simulink model "SimForcesGP2020a"  (R2020a)
settings: Solver=ode4  StartTime=0.0  StopTime=10  FixedStep=0.001  MaxStep=0.001  RelTol=1e-7
values from neighbouring files (symbols this model uses):
  B11_r_B11C = [0.23805608; 0.13201777; 0]    [InitializeSimulationGP.m]
  B11_r_B11Tc1 = [L11; 0; 0]    [InitializeSimulationGP.m]
  B11_Rot_Tc1 = eye(3)    [InitializeSimulationGP.m]
  B11cI = [0.28426000 -0.06487287 0;         -0.06487287  0.54237481 0;                   0  0          0.67891020]    [InitializeSimulationGP.m]
  B12_r_B12C = [0.60504569; 0.27199376; 0.00002484]    [InitializeSimulationGP.m]
  B12_r_B12Tc2 = [L12;0;0]    [InitializeSimulationGP.m]
  B12_Rot_Tc2 = eye(3)    [InitializeSimulationGP.m]
  B12cI = [1.18803886 -2.36786418 0.00280315;          -2.36786418 6.31493281 0.00022322;           0.00280315 0.00022322 7.40915161]    [InitializeSimulationGP.m]
  B31_r_B31C = [0.35781210 0 0]    [InitializeSimulationGP.m]
  B31_Rot_B41 = eye(3)    [InitializeSimulationGP.m]
  B31cI = diag([0.03150902 0.90735702 0.90763033])    [InitializeSimulationGP.m]
  B32_r_B32C = [0.35781210 0 0]    [InitializeSimulationGP.m]
  B32_Rot_B42 = eye(3)    [InitializeSimulationGP.m]
  B32cI = diag([0.03150902 0.90735702 0.90763033])    [InitializeSimulationGP.m]
  B41_r_B41C = [0.55785997 0 0]    [InitializeSimulationGP.m]
  B41_r_B41Tc1 = [lc1;0;0]    [InitializeSimulationGP.m]
  B41cI = diag([0.00370720 0.55759812 0.55785997])    [InitializeSimulationGP.m]
  B42_r_B42C = [0.55785997 0 0]    [InitializeSimulationGP.m]
  B42_r_B42Tc2 = [lc2; 0; 0]    [InitializeSimulationGP.m]
  B42cI = diag([0.00370720 0.55759812 0.55785997])    [InitializeSimulationGP.m]
  B52_r_B52C = [0 0 0.56802906]    [InitializeSimulationGP.m]
  B52_r_B52P32 = [lc3; 0; 0]    [InitializeSimulationGP.m]
  B52_Rot_P32 = eye(3)    [InitializeSimulationGP.m]
  B52cI = diag([0.91789884, 0.91790043, 0.00091463])    [InitializeSimulationGP.m]
  Bc1_r_Bc1B11 = [L1; 0; 0]    [InitializeSimulationGP.m]
  Bc1_r_Bc1B31 = [0;0;0]    [InitializeSimulationGP.m]
  Bc1_r_Bc1C = [0.14178771; 0.16555780; 0]    [InitializeSimulationGP.m]
  Bc1_V = [0;0;0;0;0;0]    [InitializeSimulationGP.m]
  Bc1cI = [+5.892211080 +5.476111360 -0.000019630;          +5.476111360 +28.66965601 -0.000024550;          -0.000019630 -0.000024550 +29.78955950]    [InitializeSimulationGP.m]
  Bc2_r_Bc2B12 = [L2;0;0]    [InitializeSimulationGP.m]
  Bc2_r_Bc2B32 = [0;0;0]    [InitializeSimulationGP.m]
  Bc2_r_Bc2C = [0.54319901; 0.10543875; 0]    [InitializeSimulationGP.m]
  Bc2cI = [0.48071390 0.52924041 0;          0.52924041 5.80912352 0;              0      0          5.97255351]    [InitializeSimulationGP.m]
  beta1 = atan2d(374.261,935)*pi/180    [InitializeSimulationGP.m]
  beta2 = atan2d(45.757,373.313)*pi/180    [InitializeSimulationGP.m]
  beta3 = atan2d(139.50,1132.19)*pi/180    [InitializeSimulationGP.m]
  beta4 = atan2d(88.061,296.198)*pi/180    [InitializeSimulationGP.m]
  D22F = [0;0;0;0;0;0]    [InitializeSimulationGP.m]
  L1 = 1.0071227324212    (= 1.00712273242)    [InitializeSimulationGP.m]
  L11 = 0.37610632101293    (= 0.376106321013)    [InitializeSimulationGP.m]
  L12 = 0.30901132665325    (= 0.309011326653)    [InitializeSimulationGP.m]
  L2 = 1.132185817991    (= 1.13218581799)    [InitializeSimulationGP.m]
  lc1 = 0.745    [InitializeSimulationGP.m]
  lc2 = 0.745    [InitializeSimulationGP.m]
  mB11 = 25.52660174    [InitializeSimulationGP.m]
  mB12 = 33.92850233    [InitializeSimulationGP.m]
  mB31 = 17.36281648    [InitializeSimulationGP.m]
  mB32 = 17.36281648    [InitializeSimulationGP.m]
  mB41 = 10.34519231    [InitializeSimulationGP.m]
  mB42 = 10.34519231    [InitializeSimulationGP.m]
  mB52 = 6.73059863    [InitializeSimulationGP.m]
  mBc1 = 307.29601379    [InitializeSimulationGP.m]
  mBc2 = 54.58702836    [InitializeSimulationGP.m]
  mP22 = 9.26136143    [InitializeSimulationGP.m]
  mP32 = 570.18877059    [InitializeSimulationGP.m]
  P22_r_P22C = [0.62192523 0 0]    [InitializeSimulationGP.m]
  P22_Rot_B52 = eye(3)    [InitializeSimulationGP.m]
  P22cI = diag([0.00662754, 1.48387017, 1.48398069])    [InitializeSimulationGP.m]
  P32_r_P32C = [0.25466704; -0.13034397; -0.01302248]    [InitializeSimulationGP.m]
  P32_r_P32D22 = [0.40499744871392; -0.13130517281345; -0.013385243295654]    [InitializeSimulationGP.m]
  P32_Rot_D22 = [1 0 0;              0 0.9707729441837 0.23999977258512;              0 -0.23999977258512 0.9707729441837]    [InitializeSimulationGP.m]
  P32cI = [46.81220713 0.38607676 -0.00453819;          0.38607676 71.92201786 -1.14320993;          -0.00453819 -1.14320993 67.38128576]    [InitializeSimulationGP.m]
  Tc1_r_Tc1Bc2 = [0.098495302558553; 0.01838181329939; 0]    [InitializeSimulationGP.m]
  Tc1_Rot_Bc2 = [cos(alpha2) -sin(alpha2) 0;                sin(alpha2)  cos(alpha2) 0;                0            0           1]    [InitializeSimulationGP.m]
  Tc2_r_Tc2P22 = [-0.048858374920227;0.36587359346146;0.035276938723102]    [InitializeSimulationGP.m]
  Tc2_Rot_P22 = [0.95853460763586 -0.27664713597974  0.0683942111482;                0.28497614981675  0.93051946315663 -0.23004808784757;                0                 0.23999977258511  0.9707729441837]    [InitializeSimulationGP.m]
  Th1A = 5*pi/180    (= 0.0872664625997)    [InitializeSimulationGP.m]
  Th1B = 20*pi/180    (= 0.349065850399)    [InitializeSimulationGP.m]
  Th1f = 1    [InitializeSimulationGP.m]
  Th2A = 15*pi/180    (= 0.261799387799)    [InitializeSimulationGP.m]
  Th2B = -50*pi/180    (= -0.872664625997)    [InitializeSimulationGP.m]
  Th2f = 2    [InitializeSimulationGP.m]
  W_r_WBc1 = [0.185;-0.085;0]    [InitializeSimulationGP.m]
  W_Rot_Bc1 = [cos(alpha1) -sin(alpha1) 0;              sin(alpha1)  cos(alpha1) 0;              0            0           1]    [InitializeSimulationGP.m]
  Wg = [0; 9.8066; 0]    [InitializeSimulationGP.m]
  x10 = 0.83    [InitializeSimulationGP.m]
  x20 = 0.83    [InitializeSimulationGP.m]
  x3A = 0.1    [InitializeSimulationGP.m]
  x3B = 0.5    [InitializeSimulationGP.m]
  x3f = 1    [InitializeSimulationGP.m]
  xf = [1;0;0;0;0;0]    [InitializeSimulationGP.m]
  ztau = [0;0;0;0;0;1]    [InitializeSimulationGP.m]
undefined symbols (not defined in the file or in its folder): B11_V, B11_V_SS, B11Ftot, B12_U_Tc2, B12_V, B12_V_SS, B12Ftot, B31_r_B31B41, B31_V, B31_V_SS, B31FTot, B32_r_B32B42, B32_U_B42, B32_V, B32_V_SS, B32FTot, B41_V, B41_V_SS, B41FTot, B42_Rot_Tc2, B42_U_Tc2, B42_V, B42_V_SS, B42FTot, B52_U_P32, B52_V, B52_V_SS, B52Ftot, Bc1_V_SS, Bc1Tot, Bc2_Rot_B12, Bc2_Rot_B32, Bc2_U_B12, Bc2_U_B32, Bc2_V, Bc2_V_SS, Bc2Tot, D22_V, D22_V_SS, dq1, dq11, dq12, dq2, dq21, dq22, dx1, dx2, FTot_S1, FTot_S2P, FTot_S2R, P22_r_P22B52, P22_U_B52, P22_V, P22_V_SS, P22FTot, P32_U_D22, P32_V, P32_V_SS, P32FTot, q1 ... (+28)
libraries: nesl_utility x94, sm_lib x45
(part 4 of 6)

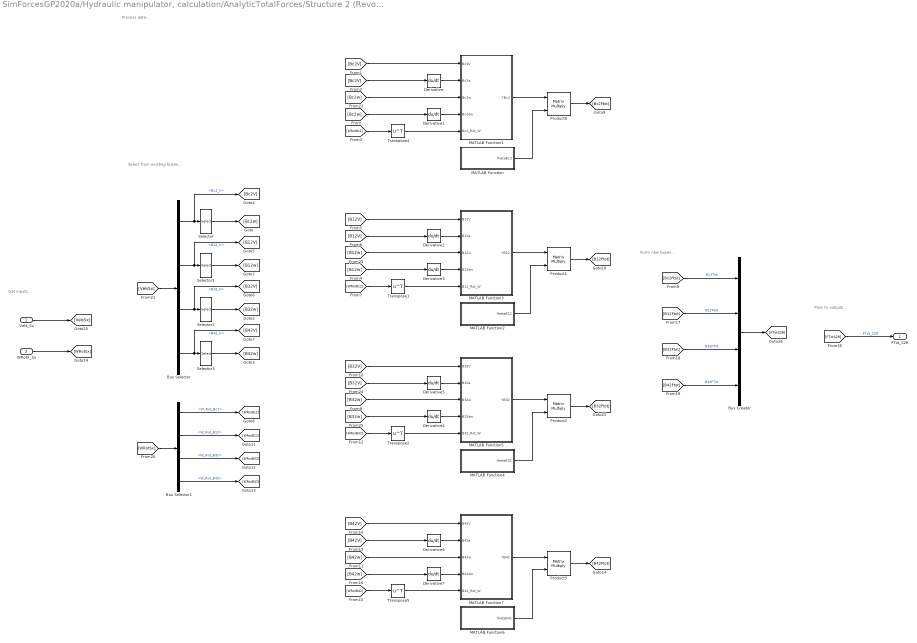
== system SimForcesGP2020a/Hydraulic manipulator, calculation/AnalyticTotalForces/Structure 2 (Revolute segment) ==
  note: Process data...
  note: Pass to outputs...
  note: Get inputs...
  note: Form new buses...
  note: Select from existing buses...
  Vels_Sx : Inport
  WRotX_Sx : Inport  Port=2
  Bus Creator : BusCreator  Inputs=Bc2Tot,B12Ftot,B32FTot,B42FTot
  Bus Selector : BusSelector  OutputSignals=Vels_S1.Bc2_V,Vels_S2R.B12_V,Vels_S2R.B32_V,Vels_S2R.B42_V
  Bus Selector1 : BusSelector  OutputSignals=WRotX_S1.W_Rot_Bc2,WRotX_S2R.W_Rot_B12,WRotX_S2R.W_Rot_B32,WRotX_S2R.W_Rot_B42
  Derivative{,1..7} (8 alike) : Derivative
  MATLAB Function : MATLAB Function  TreatAsAtomicUnit=on
  MATLAB Function1 : MATLAB Function  TreatAsAtomicUnit=on
  MATLAB Function2 : MATLAB Function  TreatAsAtomicUnit=on
  MATLAB Function3 : MATLAB Function  TreatAsAtomicUnit=on
  MATLAB Function4 : MATLAB Function  TreatAsAtomicUnit=on
  MATLAB Function5 : MATLAB Function  TreatAsAtomicUnit=on
  MATLAB Function6 : MATLAB Function  TreatAsAtomicUnit=on
  MATLAB Function7 : MATLAB Function  TreatAsAtomicUnit=on
  Product{1..3,8} (4 alike) : Product  Multiplication=Matrix(*)
  Selector{,1..3} (4 alike) : Selector  InputPortWidth=6  IndexOptions=Index vector (dialog)  Indices=[4 5 6]  OutputSizes=1
  Transpose{1..2,4..5} (4 alike) : Math  Operator=transpose  SaturateOnIntegerOverflow=on
  FTot_S2R : Outport
  wires:
  Bus Selector1/4 -> [WRotB42]  "<W_Rot_B42>"
  [WRotB12] -> Transpose1/1
  Bus Selector1/2 -> [WRotB12]  "<W_Rot_B12>"
  [WRotB42] -> Transpose5/1
  [Bc2Ftot] -> Bus Creator/1  "Bc2Tot"
  Selector2/1 -> [B32w]
  [B42Ftot] -> Bus Creator/4  "B42FTot"
  Bus Selector/2 -> Selector1/1, [B12V]  "<B12_V>"
  Bus Selector/1 -> Selector/1, [Bc2V]  "<Bc2_V>"
  [B32Ftot] -> Bus Creator/3  "B32FTot"
  Bus Selector/3 -> Selector2/1, [B32V]  "<B32_V>"
  Selector1/1 -> [B12w]
  [WRotSx] -> Bus Selector1/1
  Selector3/1 -> [B42w]
  Bus Creator/1 -> [FTotS2R]
  Selector/1 -> [Bc2w]
  [WRotB32] -> Transpose2/1
  Product3/1 -> [B42Ftot]
  Product8/1 -> [Bc2Ftot]
  [B12Ftot] -> Bus Creator/2  "B12Ftot"
  Bus Selector1/1 -> [WRotBc2]  "<W_Rot_Bc2>"
  [VelsSx] -> Bus Selector/1
  Bus Selector1/3 -> [WRotB32]  "<W_Rot_B32>"
  Bus Selector/4 -> Selector3/1, [B42V]  "<B42_V>"
  Vels_Sx/1 -> [VelsSx]
  WRotX_Sx/1 -> [WRotSx]
  [FTotS2R] -> FTot_S2R/1  "FTot_S2R"
  [Bc2w] -> Derivative1/1
  [Bc2w] -> MATLAB Function1/3(Bc2w)
  [WRotBc2] -> Transpose4/1
  Transpose4/1 -> MATLAB Function1/5(Bc2_Rot_W)
  Derivative1/1 -> MATLAB Function1/4(Bc2dw)
  [Bc2V] -> MATLAB Function1/1(Bc2V)
  MATLAB Function/1(thetaBc2) -> Product8/2
  [Bc2V] -> Derivative/1
  MATLAB Function1/1(YBc2) -> Product8/1
  Derivative/1 -> MATLAB Function1/2(Bc2a)
  Derivative2/1 -> MATLAB Function3/2(B12a)
  MATLAB Function3/1(YB12) -> Product1/1
  [B12V] -> Derivative2/1
  MATLAB Function2/1(thetaB12) -> Product1/2
  [B12V] -> MATLAB Function3/1(B12V)
  Derivative3/1 -> MATLAB Function3/4(B12dw)
  Transpose1/1 -> MATLAB Function3/5(B12_Rot_W)
  [B12w] -> MATLAB Function3/3(B12w)
  [B12w] -> Derivative3/1
  Product1/1 -> [B12Ftot]
  [B32w] -> Derivative4/1
  [B32w] -> MATLAB Function5/3(B32w)
  Derivative4/1 -> MATLAB Function5/4(B32dw)
  [B32V] -> MATLAB Function5/1(B32V)
  MATLAB Function4/1(thetaB32) -> Product2/2
  [B32V] -> Derivative5/1
  MATLAB Function5/1(YB32) -> Product2/1
  Derivative5/1 -> MATLAB Function5/2(B32a)
  Transpose2/1 -> MATLAB Function5/5(B32_Rot_W)
  Product2/1 -> [B32Ftot]
  Transpose5/1 -> MATLAB Function7/5(B42_Rot_W)
  Derivative6/1 -> MATLAB Function7/2(B42a)
  MATLAB Function7/1(YB42) -> Product3/1
  [B42V] -> Derivative6/1
  MATLAB Function6/1(thetaB42) -> Product3/2
  [B42V] -> MATLAB Function7/1(B42V)
  Derivative7/1 -> MATLAB Function7/4(B42dw)
  [B42w] -> MATLAB Function7/3(B42w)
  [B42w] -> Derivative7/1

== system SimForcesGP2020a/Hydraulic manipulator, calculation/AnalyticVelocities/Structure 1 ==
  note: Pass to outputs...
  note: Process data...
  note: Calculate geometric properties of the closed kinematic chain 1...
  note: Get inputs...
  note: Form relevant position vectors...
  note: Form relevant rotation matrices...
  note: Form relevant velocity/force transformation matrices...
  note: Form relevant linear/angular velocities...
  q1[rad] : Inport  Unit=rad
  W_Rot_Bc1 : Inport  Port=2
  Bc1_V : Inport  Port=3  PortDimensions=[6 1]
  GeomPropS1 : Subsystem
  PosVecsS1 : Subsystem
  RotMatsS1 : Subsystem
  UMatsS1 : Subsystem
  VelsS1 : Subsystem
  Geom_S1 : Outport
  PosVecs_S1 : Outport  Port=2
  WRotX_S1 : Outport  Port=3
  Vels_S1 : Outport  Port=4
  UMat_S1 : Outport  Port=5
  wires:
  GeomPropS1/1(GeomProp_S1) -> [GeomS1]
  [GeomS1] -> PosVecsS1/1(GeomProp_CC1)
  [GeomS1] -> RotMatsS1/1(GeomProp_S1)
  [GeomS1] -> VelsS1/1(GeomProp_S1)
  RotMatsS1/1(RotMats_S1) -> [RotMatsS1]
  [RotMatsS1] -> UMatsS1/2(RotMats_S1)
  PosVecsS1/1(PosVecs_S1) -> [PosVecsS1]
  [PosVecsS1] -> UMatsS1/1(PosVecs_S1)
  [GeomS1] -> Geom_S1/1
  VelsS1/1(Vels_S1) -> [VelsS1]
  [VelsS1] -> Vels_S1/1
  UMatsS1/1(UMat_S1) -> [UMatsS1]
  [UMatsS1] -> VelsS1/2(UMats_S1)
  Bc1_V/1 -> [Bc1V]  "Bc1V"
  [Bc1V] -> VelsS1/3(Bc1_V)
  W_Rot_Bc1/1 -> [WRotBc1]  "WRotBc1"
  [WRotBc1] -> RotMatsS1/2(WRotBc1)
  [UMatsS1] -> UMat_S1/1
  RotMatsS1/2(WRotX_S1) -> [WRotXS1]
  [WRotXS1] -> WRotX_S1/1
  q1[rad]/1 -> [q1]  "q1"
  [q1] -> GeomPropS1/1(q1)
  [PosVecsS1] -> PosVecs_S1/1

== system SimForcesGP2020a/Hydraulic manipulator, calculation/AnalyticVelocities/Structure 2 (Prismatic segment) ==
  note: Pass to outputs...
  note: Get inputs...
  note: Process data...
  x3 : Inport
  WRotX_S2R : Inport  Port=2
  Vels_S2R : Inport  Port=3
  GeomPropS2P : Subsystem
  PosVecsS2P : Subsystem
  RotMatsS2P : Subsystem
  UMatsS2P : Subsystem
  VelsS2P : Subsystem
  GeomProp_S2P : Outport
  PosVecs_S2P : Outport  Port=2
  WRotX_S2P : Outport  Port=3
  Vels_S2P : Outport  Port=4
  UMats_S2P : Outport  Port=5
  wires:
  x3/1 -> [x3]
  Vels_S2R/1 -> [VelsS2R]
  WRotX_S2R/1 -> [WRotXS2R]
  GeomPropS2P/1(GeomProp_S2P) -> [GeomS2P]
  [GeomS2P] -> GeomProp_S2P/1
  [x3] -> GeomPropS2P/1(x3)
  PosVecsS2P/1(PosVecsS2P) -> [PosVecsS2P]
  [x3] -> PosVecsS2P/1(x3)
  [PosVecsS2P] -> PosVecs_S2P/1
  RotMatsS2P/2(WRotX_S2P) -> [WRotXS2P]
  [WRotXS2R] -> RotMatsS2P/1(WRotX_S2R)
  [WRotXS2P] -> WRotX_S2P/1
  RotMatsS2P/1(RotMats_S2P) -> [RotMatsS2P]
  [PosVecsS2P] -> UMatsS2P/1(PosVecs_S2P)
  [RotMatsS2P] -> UMatsS2P/2(RotMats_S2P)
  UMatsS2P/1(UMats_S2P) -> [UMatsS2P]
  [UMatsS2P] -> UMats_S2P/1
  [VelsS2R] -> VelsS2P/3(Vels_S2R)
  [GeomS2P] -> VelsS2P/1(GeomProp_S2P)
  [UMatsS2P] -> VelsS2P/2(UMats_S2P)
  VelsS2P/1(Vels_S2P) -> [VelsS2P]
  [VelsS2P] -> Vels_S2P/1

== system SimForcesGP2020a/Hydraulic manipulator, calculation/AnalyticVelocities/Structure 2 (Revolute segment) ==
  note: Pass to outputs...
  note: Process data...
  note: Get inputs...
  q2[rad] : Inport
  WRotX_S1 : Inport  Port=2
  Vels_S1 : Inport  Port=3
  GeomPropS2R : Subsystem
  PosVecsS2R : Subsystem
  RotMatsS2R : Subsystem
  UMatS2R : Subsystem
  VelsS2R : Subsystem
  GeomProp_S2R : Outport
  PosVecs_S2R : Outport  Port=2
  WRotX_S2R : Outport  Port=3
  Vels_S2R : Outport  Port=4
  UMats_S2R : Outport  Port=5
  wires:
  [GeomS2R] -> VelsS2R/1(GeomProp_CC2)
  [GeomS2R] -> RotMatsS2R/1(GeomProp_CC2)
  [GeomS2R] -> PosVecsS2R/1(GeomProp_S2R)
  GeomPropS2R/1(GeomProp_S2R) -> [GeomS2R]
  [q2] -> GeomPropS2R/1(q2)
  [GeomS2R] -> GeomProp_S2R/1  "GeomS2R"
  RotMatsS2R/1(RotMats_S2) -> [RotMatsS2R]
  q2[rad]/1 -> [q2]  "q2"
  PosVecsS2R/1(PosVecs_S2) -> [PosVecsS2R]
  [PosVecsS2R] -> UMatS2R/1(PosVecs_S2)
  [PosVecsS2R] -> PosVecs_S2R/1  "PosVecsS2R"
  [RotMatsS2R] -> UMatS2R/2(RotMats_S2)
  UMatS2R/1(UMatS2) -> [UMatsS2R]
  [UMatsS2R] -> VelsS2R/2(UMats_S2)
  [UMatsS2R] -> UMats_S2R/1  "UMatsS2R"
  RotMatsS2R/2(WRotX_S2) -> [WRotXS2R]
  [WRotXS2R] -> WRotX_S2R/1  "WRotXS2R"
  Vels_S1/1 -> [VelsS1]  "Vels_S1"
  [VelsS1] -> VelsS2R/3(Vels_S1)
  WRotX_S1/1 -> [WRotXS1]  "WRotX_S1"
  [WRotXS1] -> RotMatsS2R/2(WRotX_S1)
  VelsS2R/1(Vels_S2) -> [VelsS2R]
  [VelsS2R] -> Vels_S2R/1  "VelsS2R"

== system SimForcesGP2020a/Hydraulic manipulator, calculation/AnalyticVelocities/Structure 1/GeomPropS1 ==
  note: Get inputs...
  note: Pass to outputs...
  note: Process data...
  note: Create new buses...
  q1 : Inport
  Bus Creator : BusCreator  Inputs=q1,x1,q11,q12,dq1,dx1,dq11,dq12
  LiftPistonStroke : Subsystem
  Subsystem : Subsystem
  Subsystem1 : Subsystem
  Subsystem2 : Subsystem
  q11-angle : Subsystem
  q12-angle : Subsystem
  q1Derivative : Subsystem
  GeomProp_S1 : Outport
  wires:
  q1/1 -> [q1]  "q1"
  [q1] -> LiftPistonStroke/1(q1[rad])  "q1"
  LiftPistonStroke/1(x1[m]) -> [x1]  "x1"
  [x1] -> q11-angle/1(x1)  "x1"
  [x1] -> q12-angle/1(x1)  "x1"
  [dq1] -> Bus Creator/5  "dq1"
  q12-angle/1(q12) -> [q12]  "q12"
  [q12] -> Bus Creator/4  "q12"
  [q1] -> Bus Creator/1  "q1"
  [x1] -> Bus Creator/2  "x1"
  q11-angle/1(q11) -> [q11]  "q11"
  [q11] -> Bus Creator/3  "q11"
  [dx1] -> Bus Creator/6  "dx1"
  [dq12] -> Bus Creator/8  "dq12"
  [dq11] -> Bus Creator/7  "dq11"
  Bus Creator/1 -> [GeomPropS1]
  [GeomPropS1] -> GeomProp_S1/1
  [q1] -> q1Derivative/1(q1)  "q1"
  q1Derivative/1(dq1) -> [dq1]  "dq1"
  [dq1] -> Subsystem/1(dq1)  "dq1"
  [x1] -> Subsystem/2(x1)  "x1"
  [q1] -> Subsystem/3(q1)  "q1"
  Subsystem/1(dx1) -> [dx1]  "dx1"
  [dx1] -> Subsystem1/3(dx1)  "dx1"
  [x1] -> Subsystem1/1(x1)  "x1"
  [q11] -> Subsystem1/2(q11)  "q11"
  Subsystem1/1(dq11) -> [dq11]  "dq11"
  Subsystem2/1(dq12) -> [dq12]  "dq12"
  [dx1] -> Subsystem2/3(dx1)  "dx1"
  [x1] -> Subsystem2/1(x1)  "x1"
  [q12] -> Subsystem2/2(q12)  "q12"

== system SimForcesGP2020a/Hydraulic manipulator, calculation/AnalyticVelocities/Structure 1/PosVecsS1 ==
  note: Select from existing buses...
  note: Pass to outputs...
  note: Create new buses...
  note: Process data...
  note: Form time-varying position vectors...
  note: Get inputs...
  GeomProp_CC1 : Inport
  B11_r_B11Tc1 : Constant  Value=B11_r_B11Tc1
  B31_r_B31B41 : MATLAB Function  TreatAsAtomicUnit=on
  B41_r_B41Tc1 : Constant  Value=B41_r_B41Tc1
  Bc1_r_Bc1B1 : Constant  Value=W_r_WBc1
  Bc1_r_Bc1B11 : Constant  Value=Bc1_r_Bc1B11
  Bc1_r_Bc1B31 : Constant  Value=Bc1_r_Bc1B31
  Bus Creator : BusCreator  Inputs=Tc1_r_Tc1Bc2,B41_r_B41Tc1,B31_r_B31B41,Bc1_r_Bc1B31,B11_r_B11Tc1,Bc1_r_Bc1B11,W_r_WBc1
  Bus Selector : BusSelector  OutputSignals=x1
  Tc1_r_Tc1Bc2 : Constant  Value=Tc1_r_Tc1Bc2
  PosVecs_S1 : Outport
  wires:
  Bus Creator/1 -> [PosVecsS1]
  GeomProp_CC1/1 -> [GeomPropCC1]  "GeomProp_CC1"
  [GeomPropCC1] -> Bus Selector/1
  Tc1_r_Tc1Bc2/1 -> [rTc1Bc2]  "Tc1_r_Tc1Bc2"
  [rTc1Bc2] -> Bus Creator/1  "Tc1_r_Tc1Bc2"
  B41_r_B41Tc1/1 -> [rB41Tc1]  "B41_r_B41Tc1"
  [rB41Tc1] -> Bus Creator/2  "B41_r_B41Tc1"
  B31_r_B31B41/1(B31_r_B31B41) -> [rB31B41]  "B31_r_B31B41"
  [rB31B41] -> Bus Creator/3  "B31_r_B31B41"
  Bc1_r_Bc1B31/1 -> [rBc1B31]  "Bc1_r_Bc1B31"
  B11_r_B11Tc1/1 -> [rB11Tc1]  "B11_r_B11Tc1"
  Bc1_r_Bc1B11/1 -> [rBc1B11]  "Bc1_r_Bc1B11"
  [rBc1B31] -> Bus Creator/4  "Bc1_r_Bc1B31"
  [rB11Tc1] -> Bus Creator/5  "B11_r_B11Tc1"
  [rBc1B11] -> Bus Creator/6  "Bc1_r_Bc1B11"
  Bus Selector/1 -> [x1]  "<x1>"
  [x1] -> B31_r_B31B41/1(x1)
  [PosVecsS1] -> PosVecs_S1/1  "PosVecs_S1"
  [rWBc1] -> Bus Creator/7  "W_r_WBc1"
  Bc1_r_Bc1B1/1 -> [rWBc1]  "W_r_WBc1"

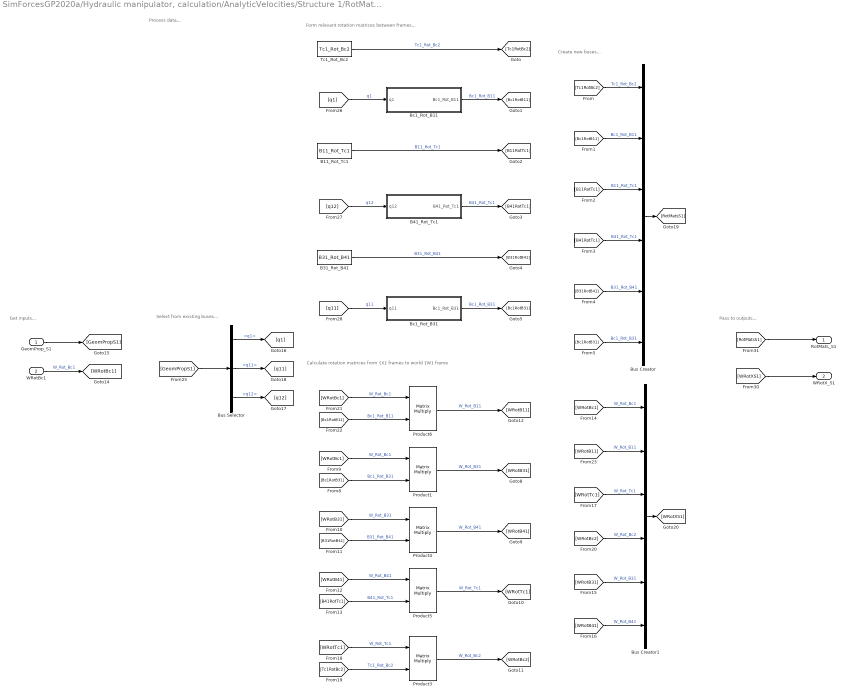
== system SimForcesGP2020a/Hydraulic manipulator, calculation/AnalyticVelocities/Structure 1/RotMatsS1 ==
  note: Create new buses...
  note: Pass to outputs...
  note: Get inputs...
  note: Process data...
  note: Select from existing buses...
  note: Form relevant rotation matrices between frames...
  note: Calculate rotation matrices from {X} frames to world {W} frame
  GeomProp_S1 : Inport
  WRotBc1 : Inport  Port=2
  B11_Rot_Tc1 : Constant  Value=B11_Rot_Tc1
  B31_Rot_B41 : Constant  Value=B31_Rot_B41
  B41_Rot_Tc1 : MATLAB Function  TreatAsAtomicUnit=on
  Bc1_Rot_B11 : MATLAB Function  TreatAsAtomicUnit=on
  Bc1_Rot_B31 : MATLAB Function  TreatAsAtomicUnit=on
  Bus Creator : BusCreator  Inputs=6
  Bus Creator1 : BusCreator  Inputs=W_Rot_Bc1,W_Rot_B11,W_Rot_Tc1,W_Rot_Bc2,W_Rot_B31,W_Rot_B41
  Bus Selector : BusSelector  OutputSignals=q1,q11,q12
  Product{1,3..6} (5 alike) : Product  Multiplication=Matrix(*)
  Tc1_Rot_Bc2 : Constant  Value=Tc1_Rot_Bc2
  RotMats_S1 : Outport
  WRotX_S1 : Outport  Port=2
  wires:
  [Tc1RotBc2] -> Bus Creator/1  "Tc1_Rot_Bc2"
  Tc1_Rot_Bc2/1 -> [Tc1RotBc2]  "Tc1_Rot_Bc2"
  [Bc1RotB11] -> Bus Creator/2  "Bc1_Rot_B11"
  Bc1_Rot_B11/1(Bc1_Rot_B11) -> [Bc1RotB11]  "Bc1_Rot_B11"
  [B11RotTc1] -> Bus Creator/3  "B11_Rot_Tc1"
  B11_Rot_Tc1/1 -> [B11RotTc1]  "B11_Rot_Tc1"
  B41_Rot_Tc1/1(B41_Rot_Tc1) -> [B41RotTc1]  "B41_Rot_Tc1"
  [B41RotTc1] -> Bus Creator/4  "B41_Rot_Tc1"
  B31_Rot_B41/1 -> [B31RotB41]  "B31_Rot_B41"
  [B31RotB41] -> Bus Creator/5  "B31_Rot_B41"
  Bc1_Rot_B31/1(Bc1_Rot_B31) -> [Bc1RotB31]  "Bc1_Rot_B31"
  [Bc1RotB31] -> Bus Creator/6  "Bc1_Rot_B31"
  [WRotBc1] -> Product1/1  "W_Rot_Bc1"
  [Bc1RotB31] -> Product1/2  "Bc1_Rot_B31"
  Product1/1 -> [WRotB31]  "W_Rot_B31"
  [WRotB31] -> Product4/1  "W_Rot_B31"
  [B31RotB41] -> Product4/2  "B31_Rot_B41"
  Product4/1 -> [WRotB41]  "W_Rot_B41"
  Product5/1 -> [WRotTc1]  "W_Rot_Tc1"
  [B41RotTc1] -> Product5/2  "B41_Rot_Tc1"
  [WRotB41] -> Product5/1  "W_Rot_B41"
  [WRotTc1] -> Product3/1  "W_Rot_Tc1"
  [Tc1RotBc2] -> Product3/2  "Tc1_Rot_Bc2"
  Product3/1 -> [WRotBc2]  "W_Rot_Bc2"
  [WRotBc1] -> Product6/1  "W_Rot_Bc1"
  [Bc1RotB11] -> Product6/2  "Bc1_Rot_B11"
  Product6/1 -> [WRotB11]  "W_Rot_B11"
  [WRotB11] -> Bus Creator1/2  "W_Rot_B11"
  [WRotBc1] -> Bus Creator1/1  "W_Rot_Bc1"
  [WRotB41] -> Bus Creator1/6  "W_Rot_B41"
  [WRotB31] -> Bus Creator1/5  "W_Rot_B31"
  [WRotBc2] -> Bus Creator1/4  "W_Rot_Bc2"
  [WRotTc1] -> Bus Creator1/3  "W_Rot_Tc1"
  WRotBc1/1 -> [WRotBc1]  "W_Rot_Bc1"
  GeomProp_S1/1 -> [GeomPropS1]
  [GeomPropS1] -> Bus Selector/1
  Bus Selector/1 -> [q1]  "<q1>"
  Bus Selector/3 -> [q12]  "<q12>"
  Bus Selector/2 -> [q11]  "<q11>"
  [q1] -> Bc1_Rot_B11/1(q1)  "q1"
  [q12] -> B41_Rot_Tc1/1(q12)  "q12"
  [q11] -> Bc1_Rot_B31/1(q11)  "q11"
  Bus Creator/1 -> [RotMatsS1]
  Bus Creator1/1 -> [WRotXS1]
  [WRotXS1] -> WRotX_S1/1
  [RotMatsS1] -> RotMats_S1/1

== system SimForcesGP2020a/Hydraulic manipulator, calculation/AnalyticVelocities/Structure 1/UMatsS1 ==
  note: Get inputs...
  note: Pass to outputs...
  note: Form new buses...
  note: Process data...
  note: Form relevant velocity/force transformation matrices...
  note: Select form existing buses...
  PosVecs_S1 : Inport
  RotMats_S1 : Inport  Port=2
  B11_U_Tc1 : MATLAB Function  TreatAsAtomicUnit=on
  B31_U_B41 : MATLAB Function  TreatAsAtomicUnit=on
  B41_U_Tc1 : MATLAB Function  TreatAsAtomicUnit=on
  Bc1_U_B11 : MATLAB Function  TreatAsAtomicUnit=on
  Bc1_U_B31 : MATLAB Function  TreatAsAtomicUnit=on
  Bus Creator : BusCreator  Inputs=6
  Bus Selector : BusSelector  OutputSignals=Tc1_r_Tc1Bc2,B41_r_B41Tc1,B31_r_B31B41,Bc1_r_Bc1B31,B11_r_B11Tc1,Bc1_r_Bc1B11
  Bus Selector1 : BusSelector  OutputSignals=Tc1_Rot_Bc2,B41_Rot_Tc1,B31_Rot_B41,Bc1_Rot_B31,B11_Rot_Tc1,Bc1_Rot_B11
  Tc1_U_Bc2 : MATLAB Function  TreatAsAtomicUnit=on
  UMat_S1 : Outport
  wires:
  Bus Selector/2 -> [rB41Tc1]  "<B41_r_B41Tc1>"
  [rB41Tc1] -> B41_U_Tc1/1(B41_r_B41Tc1)
  Bus Selector/3 -> [rB31B41]  "<B31_r_B31B41>"
  Bus Selector/5 -> [rB11Tc1]  "<B11_r_B11Tc1>"
  Bus Selector/4 -> [rBc1B31]  "<Bc1_r_Bc1B31>"
  Bus Selector/6 -> [rBc1B11]  "<Bc1_r_Bc1B11>"
  [rBc1B11] -> Bc1_U_B11/1(Bc1_r_Bc1B11)
  [rB11Tc1] -> B11_U_Tc1/1(B11_r_B11Tc1)
  [rBc1B31] -> Bc1_U_B31/1(Bc1_r_Bc1B31)
  [rB31B41] -> B31_U_B41/1(B31_r_B31B41)
  Bus Selector1/2 -> [B41RotTc1]  "<B41_Rot_Tc1>"
  Bus Selector1/3 -> [B31RotB41]  "<B31_Rot_B41>"
  Bus Selector1/4 -> [Bc1RotB31]  "<Bc1_Rot_B31>"
  Bus Selector1/5 -> [B11RotTc1]  "<B11_Rot_Tc1>"
  Bus Selector1/6 -> [Bc1RotB11]  "<Bc1_Rot_B11>"
  [Bc1RotB11] -> Bc1_U_B11/2(Bc1_Rot_B11)
  [B11RotTc1] -> B11_U_Tc1/2(B11_Rot_Tc1)
  [Bc1RotB31] -> Bc1_U_B31/2(Bc1_Rot_B31)
  [B31RotB41] -> B31_U_B41/2(B31_Rot_B41)
  [B41RotTc1] -> B41_U_Tc1/2(B41_Rot_Tc1)
  Bus Selector1/1 -> [Tc1RotBc2]  "<Tc1_Rot_Bc2>"
  Bus Selector/1 -> [rTc1Bc2]  "<Tc1_r_Tc1Bc2>"
  [Tc1RotBc2] -> Tc1_U_Bc2/2(Tc1_Rot_Bc2)
  [rTc1Bc2] -> Tc1_U_Bc2/1(Tc1_r_Tc1Bc2)
  Bus Creator/1 -> [UMatS1]  "UMat_S1"
  PosVecs_S1/1 -> [PosVecsS1]
  [PosVecsS1] -> Bus Selector/1
  RotMats_S1/1 -> [RotMatsS1]
  [RotMatsS1] -> Bus Selector1/1
  Tc1_U_Bc2/1(Tc1_U_Bc2) -> [Tc1UBc2]  "Tc1_U_Bc2"
  [Tc1UBc2] -> Bus Creator/1  "Tc1_U_Bc2"
  B41_U_Tc1/1(B41_U_Tc1) -> [B41UTc1]  "B41_U_Tc1"
  [B41UTc1] -> Bus Creator/2  "B41_U_Tc1"
  B31_U_B41/1(B31_U_B41) -> [B31UB41]  "B31_U_B41"
  [B31UB41] -> Bus Creator/3  "B31_U_B41"
  Bc1_U_B31/1(Bc1_U_B31) -> [Bc1UB31]  "Bc1_U_B31"
  B11_U_Tc1/1(B11_U_Tc1) -> [B11UTc1]  "B11_U_Tc1"
  Bc1_U_B11/1(Bc1_U_B11) -> [Bc1UB11]  "Bc1_U_B11"
  [Bc1UB31] -> Bus Creator/4  "Bc1_U_B31"
  [B11UTc1] -> Bus Creator/5  "B11_U_Tc1"
  [Bc1UB11] -> Bus Creator/6  "Bc1_U_B11"
  [UMatS1] -> UMat_S1/1

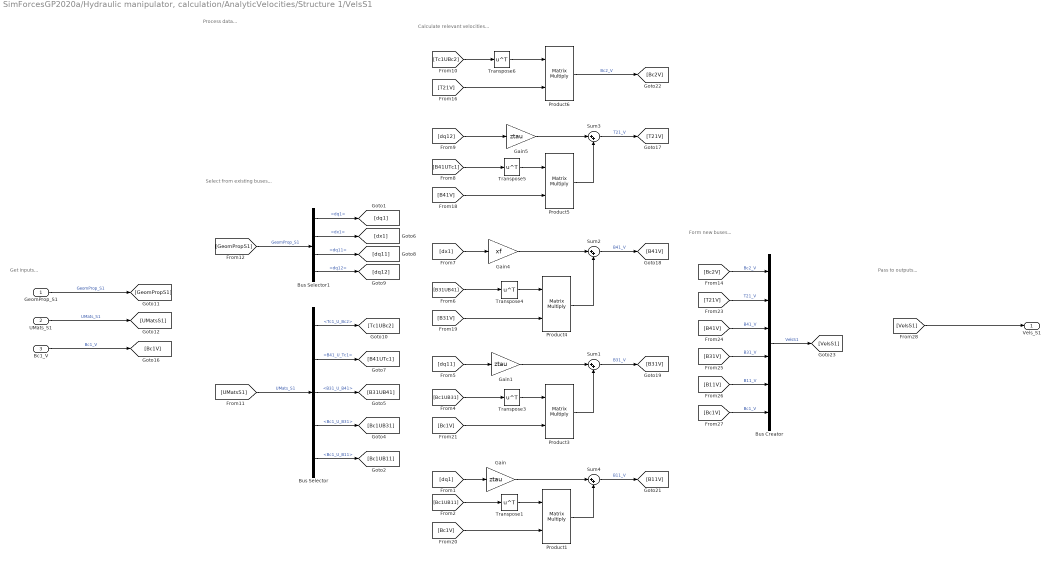
== system SimForcesGP2020a/Hydraulic manipulator, calculation/AnalyticVelocities/Structure 1/VelsS1 ==
  note: Process data...
  note: Pass to outputs...
  note: Form new buses...
  note: Calculate relevant velocities...
  note: Select from existing buses...
  note: Get inputs...
  GeomProp_S1 : Inport
  UMats_S1 : Inport  Port=2
  Bc1_V : Inport  Port=3
  Bus Creator : BusCreator  Inputs=Bc2_V,T21_V,B41_V,B31_V,B11_V,Bc1_V
  Bus Selector : BusSelector  OutputSignals=Tc1_U_Bc2,B41_U_Tc1,B31_U_B41,Bc1_U_B31,Bc1_U_B11
  Bus Selector1 : BusSelector  OutputSignals=dq1,dx1,dq11,dq12
  Gain : Gain  Gain=ztau
  Gain1 : Gain  Gain=ztau
  Gain4 : Gain  Gain=xf
  Gain5 : Gain  Gain=ztau
  Product{1,3..6} (5 alike) : Product  Multiplication=Matrix(*)
  Sum{1..4} (4 alike) : Sum  Inputs=|++
  Transpose{1,3..6} (5 alike) : Math  Operator=transpose  SaturateOnIntegerOverflow=on
  Vels_S1 : Outport
  wires:
  Product1/1 -> Sum4/2
  Gain1/1 -> Sum1/1
  Gain5/1 -> Sum3/1
  Gain/1 -> Sum4/1
  Product4/1 -> Sum2/2
  Gain4/1 -> Sum2/1
  Product5/1 -> Sum3/2
  Transpose1/1 -> Product1/1
  Bus Selector1/1 -> [dq1]  "<dq1>"
  [dq1] -> Gain/1
  Bus Selector/5 -> [Bc1UB11]  "<Bc1_U_B11>"
  [Bc1UB11] -> Transpose1/1
  Bus Selector/4 -> [Bc1UB31]  "<Bc1_U_B31>"
  Transpose3/1 -> Product3/1
  [Bc1UB31] -> Transpose3/1
  Product3/1 -> Sum1/2
  [dq11] -> Gain1/1
  Bus Selector/3 -> [B31UB41]  "<B31_U_B41>"
  Transpose4/1 -> Product4/1
  [B31UB41] -> Transpose4/1
  Bus Selector1/2 -> [dx1]  "<dx1>"
  [dx1] -> Gain4/1
  Bus Selector/2 -> [B41UTc1]  "<B41_U_Tc1>"
  [B41UTc1] -> Transpose5/1
  Transpose5/1 -> Product5/1
  Bus Selector1/4 -> [dq12]  "<dq12>"
  Bus Selector1/3 -> [dq11]  "<dq11>"
  [dq12] -> Gain5/1
  Bus Selector/1 -> [Tc1UBc2]  "<Tc1_U_Bc2>"
  [Tc1UBc2] -> Transpose6/1
  Transpose6/1 -> Product6/1
  GeomProp_S1/1 -> [GeomPropS1]  "GeomProp_S1"
  UMats_S1/1 -> [UMatsS1]  "UMats_S1"
  [UMatsS1] -> Bus Selector/1  "UMats_S1"
  [GeomPropS1] -> Bus Selector1/1  "GeomProp_S1"
  Bc1_V/1 -> [Bc1V]  "Bc1_V"
  [T21V] -> Product6/2
  Sum3/1 -> [T21V]  "T21_V"
  Sum2/1 -> [B41V]  "B41_V"
  [B41V] -> Product5/2
  Sum1/1 -> [B31V]  "B31_V"
  [B31V] -> Product4/2
  [Bc1V] -> Product1/2
  [Bc1V] -> Product3/2
  Sum4/1 -> [B11V]  "B11_V"
  Product6/1 -> [Bc2V]  "Bc2_V"
  [Bc2V] -> Bus Creator/1  "Bc2_V"
  [T21V] -> Bus Creator/2  "T21_V"
  [B41V] -> Bus Creator/3  "B41_V"
  [B31V] -> Bus Creator/4  "B31_V"
  [B11V] -> Bus Creator/5  "B11_V"
  [Bc1V] -> Bus Creator/6  "Bc1_V"
  Bus Creator/1 -> [VelsS1]  "VelsS1"
  [VelsS1] -> Vels_S1/1

== system SimForcesGP2020a/Hydraulic manipulator, calculation/AnalyticVelocities/Structure 2 (Prismatic segment)/GeomPropS2P ==
  note: Pass to outputs...
  note: Process data...
  note: Get inputs...
  x3 : Inport
  Bus Creator : BusCreator  Inputs=1
  Derivative4 : Derivative
  GeomProp_S2P : Outport
  wires:
  x3/1 -> [x3]
  [x3] -> Derivative4/1
  Derivative4/1 -> [dx3]
  [dx3] -> Bus Creator/1  "dx3"
  Bus Creator/1 -> GeomProp_S2P/1

== system SimForcesGP2020a/Hydraulic manipulator, calculation/AnalyticVelocities/Structure 2 (Prismatic segment)/PosVecsS2P ==
  note: Pass to outputs...
  note: Process data...
  note: Get inputs...
  x3 : Inport
  Bus Creator : BusCreator  Inputs=P22_r_P22B52,B52_r_B52P32,P32_r_P32D22
  Constant : Constant  Value=B52_r_B52P32
  Constant1 : Constant  Value=P32_r_P32D22
  P22_r_P22B52 : MATLAB Function  TreatAsAtomicUnit=on
  PosVecsS2P : Outport
  wires:
  x3/1 -> [x3]
  [x3] -> P22_r_P22B52/1(x3)
  P22_r_P22B52/1(P22_r_P22B52) -> [rP22B52]  "P22_r_P22B52"
  Constant/1 -> [rB52P32]  "B52_r_B52P32"
  [rP22B52] -> Bus Creator/1  "P22_r_P22B52"
  [rB52P32] -> Bus Creator/2  "B52_r_B52P32"
  Bus Creator/1 -> [PosVecsS2P]
  [PosVecsS2P] -> PosVecsS2P/1
  Constant1/1 -> [rP32D22]  "P32_r_P32D22"
  [rP32D22] -> Bus Creator/3  "P32_r_P32D22"

== system SimForcesGP2020a/Hydraulic manipulator, calculation/AnalyticVelocities/Structure 2 (Prismatic segment)/RotMatsS2P ==
  note: Pass to outputs...
  note: Get inputs...
  note: Process data...
  WRotX_S2R : Inport
  Bus Creator1 : BusCreator  Inputs=W_Rot_B52,W_Rot_P32,W_Rot_D22
  Bus Creator2 : BusCreator  Inputs=P22_Rot_B52,B52_Rot_P32,P32_Rot_D22
  Bus Selector : BusSelector  OutputSignals=W_Rot_P22
  Constant : Constant  Value=P22_Rot_B52
  Constant1 : Constant  Value=B52_Rot_P32
  Constant2 : Constant  Value=P32_Rot_D22
  Product : Product  Multiplication=Matrix(*)
  Product1 : Product  Multiplication=Matrix(*)
  Product2 : Product  Multiplication=Matrix(*)
  RotMats_S2P : Outport
  WRotX_S2P : Outport  Port=2
  wires:
  Constant/1 -> [P22RotB52]  "P22_Rot_B52"
  Constant1/1 -> [B52RotP32]  "B52_Rot_P32"
  [WRotP22] -> Product/1
  [P22RotB52] -> Product/2
  Product/1 -> [WRotB52]
  [B52RotP32] -> Product1/2
  [WRotB52] -> Product1/1
  Product1/1 -> [WRotP32]
  [WRotB52] -> Bus Creator1/1  "W_Rot_B52"
  [WRotP32] -> Bus Creator1/2  "W_Rot_P32"
  [B52RotP32] -> Bus Creator2/2  "B52_Rot_P32"
  [P22RotB52] -> Bus Creator2/1  "P22_Rot_B52"
  Bus Selector/1 -> [WRotP22]  "<W_Rot_P22>"
  WRotX_S2R/1 -> [WRotXS2R]
  [WRotXS2R] -> Bus Selector/1
  Bus Creator2/1 -> [RotMatsS2P]  "RotMats_Ext1"
  Bus Creator1/1 -> [WRotXS2P]
  [WRotXS2P] -> WRotX_S2P/1
  [RotMatsS2P] -> RotMats_S2P/1
  Constant2/1 -> [P32RotD22]  "P32_Rot_D22"
  [WRotP32] -> Product2/1
  [P32RotD22] -> Product2/2
  [P32RotD22] -> Bus Creator2/3  "P32_Rot_D22"
  [WRotD22] -> Bus Creator1/3  "W_Rot_D22"
  Product2/1 -> [WRotD22]

== system SimForcesGP2020a/Hydraulic manipulator, calculation/AnalyticVelocities/Structure 2 (Prismatic segment)/UMatsS2P ==
  note: Pass to outputs...
  note: Process data...
  note: Get inputs...
  PosVecs_S2P : Inport
  RotMats_S2P : Inport  Port=2
  B52_U_P32 : MATLAB Function  TreatAsAtomicUnit=on
  Bus Creator : BusCreator  Inputs=P22_U_B52,B52_U_P32,P32_U_D22
  Bus Selector : BusSelector  OutputSignals=P22_r_P22B52,B52_r_B52P32,P32_r_P32D22
  Bus Selector1 : BusSelector  OutputSignals=P22_Rot_B52,B52_Rot_P32,P32_Rot_D22
  P22_U_B52 : MATLAB Function  TreatAsAtomicUnit=on
  P32_U_D22 : MATLAB Function  TreatAsAtomicUnit=on
  UMats_S2P : Outport
  wires:
  PosVecs_S2P/1 -> [PosVecsS2P]
  RotMats_S2P/1 -> [RotMatsS2P]
  [PosVecsS2P] -> Bus Selector/1
  [RotMatsS2P] -> Bus Selector1/1
  Bus Selector/1 -> [rP22B52]  "<P22_r_P22B52>"
  Bus Selector1/1 -> [P22RotB52]  "<P22_Rot_B52>"
  Bus Selector1/2 -> [B52RotP32]  "<B52_Rot_P32>"
  Bus Selector/2 -> [rB52P32]  "<B52_r_B52P32>"
  [rP22B52] -> P22_U_B52/1(P22_r_P22B52)
  [P22RotB52] -> P22_U_B52/2(P22_Rot_B52)
  P22_U_B52/1(P22_U_B52) -> [P22UB52]  "P22_U_B52"
  [B52RotP32] -> B52_U_P32/2(B52_Rot_B32)
  [rB52P32] -> B52_U_P32/1(B52_r_B52B32)
  B52_U_P32/1(B52_U_P32) -> [B52UP32]  "B52_U_P32"
  [P22UB52] -> Bus Creator/1  "P22_U_B52"
  [B52UP32] -> Bus Creator/2  "B52_U_P32"
  [UMatsS2P] -> UMats_S2P/1
  Bus Creator/1 -> [UMatsS2P]
  Bus Selector1/3 -> [P32RotD22]  "<P32_Rot_D22>"
  Bus Selector/3 -> [rP32D22]  "<P32_r_P32D22>"
  [rP32D22] -> P32_U_D22/1(P32_r_P32D22)
  [P32RotD22] -> P32_U_D22/2(P32_Rot_D22)
  P32_U_D22/1(P32_U_D22) -> [P32UD22]  "P32_U_D22"
  [P32UD22] -> Bus Creator/3  "P32_U_D22"

== system SimForcesGP2020a/Hydraulic manipulator, calculation/AnalyticVelocities/Structure 2 (Prismatic segment)/VelsS2P ==
  note: Pass to outputs...
  note: Process data...
  note: Get inputs...
  GeomProp_S2P : Inport
  UMats_S2P : Inport  Port=2
  Vels_S2R : Inport  Port=3
  Bus Creator : BusCreator  Inputs=B52_V,P32_V,D22_V
  Bus Selector : BusSelector  OutputSignals=dx3
  Bus Selector1 : BusSelector  OutputSignals=P22_V
  Bus Selector2 : BusSelector  OutputSignals=P22_U_B52,B52_U_P32,P32_U_D22
  Gain : Gain  Gain=xf
  Product : Product  Multiplication=Matrix(*)
  Product1 : Product  Multiplication=Matrix(*)
  Product2 : Product  Multiplication=Matrix(*)
  Sum : Sum  Inputs=|++
  Transpose : Math  Operator=transpose  SaturateOnIntegerOverflow=on
  Transpose1 : Math  Operator=transpose  SaturateOnIntegerOverflow=on
  Transpose2 : Math  Operator=transpose  SaturateOnIntegerOverflow=on
  Vels_S2P : Outport
  wires:
  GeomProp_S2P/1 -> [GeomS2P]
  Vels_S2R/1 -> [VelsS2R]
  [GeomS2P] -> Bus Selector/1
  [VelsS2R] -> Bus Selector1/1
  UMats_S2P/1 -> [UMatsS2P]
  Bus Selector/1 -> [dx3]  "<dx3>"
  Bus Selector1/1 -> [P22V]  "<P22_V>"
  [dx3] -> Gain/1
  Sum/1 -> [B52V]
  [UMatsS2P] -> Bus Selector2/1
  Bus Selector2/1 -> [P22UB52]  "<P22_U_B52>"
  Bus Selector2/2 -> [B52UP32]  "<B52_U_P32>"
  Gain/1 -> Sum/1
  Product/1 -> Sum/2
  [P22V] -> Product/2
  [P22UB52] -> Transpose/1
  Transpose/1 -> Product/1
  [B52V] -> Product1/2
  Transpose1/1 -> Product1/1
  [B52UP32] -> Transpose1/1
  Product1/1 -> [P32V]
  [P32V] -> Bus Creator/2  "P32_V"
  [B52V] -> Bus Creator/1  "B52_V"
  Bus Creator/1 -> [VelsS2P]
  [VelsS2P] -> Vels_S2P/1
  Bus Selector2/3 -> [P32UG]  "<P32_U_D22>"
  [P32V] -> Product2/2
  [P32UG] -> Transpose2/1
  Transpose2/1 -> Product2/1
  Product2/1 -> [D22V]
  [D22V] -> Bus Creator/3  "D22_V"

== system SimForcesGP2020a/Hydraulic manipulator, calculation/AnalyticVelocities/Structure 2 (Revolute segment)/GeomPropS2R ==
  note: Pass to outputs...
  note: Process data...
  note: Get inputs...
  q2 : Inport
  Bus Creator : BusCreator  Inputs=q2,x2,q21,q22,dq2,dx2,dq21,dq22
  Subsystem4 : Subsystem
  Subsystem5 : Subsystem
  TiltPistonStroke : Subsystem
  TiltPistonVelocity : Subsystem
  q21-angle : Subsystem
  q22-angle : Subsystem
  q2Derivative : Subsystem
  GeomProp_S2R : Outport
  wires:
  q2/1 -> [q2]  "q2"
  [q2] -> TiltPistonStroke/1(q2[rad])  "q2"
  TiltPistonStroke/1(x2[m]) -> [x2]  "x2"
  [x2] -> q21-angle/1(x2)  "x2"
  [x2] -> q22-angle/1(x2)  "x2"
  [dq2] -> Bus Creator/5  "dq2"
  q21-angle/1(q21) -> [q21]  "q21"
  [q21] -> Bus Creator/3  "q21"
  [q2] -> Bus Creator/1  "q2"
  [x2] -> Bus Creator/2  "x2"
  [dx2] -> Bus Creator/6  "dx2"
  q22-angle/1(q22) -> [q22]  "q22"
  [q22] -> Bus Creator/4  "q22"
  Subsystem4/1(dq21) -> [dq21]  "dq21"
  [dq21] -> Bus Creator/7  "dq21"
  [dq22] -> Bus Creator/8  "dq22"
  q2Derivative/1(dq2) -> [dq2]  "dq2"
  [q2] -> q2Derivative/1(q2)  "q2"
  TiltPistonVelocity/1(dx2) -> [dx2]  "dx2"
  [dq2] -> TiltPistonVelocity/1(dq2)  "dq2"
  [x2] -> TiltPistonVelocity/2(x2)  "x2"
  [q2] -> TiltPistonVelocity/3(q2)  "q2"
  Bus Creator/1 -> [GeomS2R]
  [GeomS2R] -> GeomProp_S2R/1  "GeomProp_S2R"
  [x2] -> Subsystem4/1(x2)  "x2"
  [q21] -> Subsystem4/2(q21)  "q21"
  [dx2] -> Subsystem4/3(dx2)  "dx2"
  Subsystem5/1(dq22) -> [dq22]  "dq22"
  [x2] -> Subsystem5/1(x2)  "x2"
  [q22] -> Subsystem5/2(q22)  "q22"
  [dx2] -> Subsystem5/3(dx2)  "dx2"

== system SimForcesGP2020a/Hydraulic manipulator, calculation/AnalyticVelocities/Structure 2 (Revolute segment)/PosVecsS2R ==
  note: Pass to outputs...
  note: Process data...
  note: Get inputs...
  GeomProp_S2R : Inport
  B12_r_B12Tc2 : Constant  Value=B12_r_B12Tc2
  B32_r_B32B42 : MATLAB Function  TreatAsAtomicUnit=on
  B42_r_B42Tc2 : Constant  Value=B42_r_B42Tc2
  Bc2_r_Bc2B12 : Constant  Value=Bc2_r_Bc2B12
  Bc2_r_Bc2B32 : Constant  Value=Bc2_r_Bc2B32
  Bus Creator : BusCreator  Inputs=Tc2_r_Tc2P22,B42_r_B42Tc2,B32_r_B32B42,Bc2_r_Bc2B32,B12_r_B12Tc2,Bc2_r_Bc2B12
  Bus Selector : BusSelector  OutputSignals=x2
  Tc2_r_Tc2P22 : Constant  Value=Tc2_r_Tc2P22
  PosVecs_S2 : Outport
  wires:
  Bus Selector/1 -> B32_r_B32B42/1(x2)  "<x2>"
  GeomProp_S2R/1 -> [GeomPropS2R]
  [GeomPropS2R] -> Bus Selector/1
  Tc2_r_Tc2P22/1 -> [rTc2P22]  "Tc2_r_Tc2P22"
  B42_r_B42Tc2/1 -> [rB42Tc2]  "B42_r_B42Tc2"
  B32_r_B32B42/1(B32_r_B32B42) -> [rB32B42]  "B32_r_B32B42"
  Bc2_r_Bc2B32/1 -> [rBc2B32]  "Bc2_r_Bc2B32"
  B12_r_B12Tc2/1 -> [rB12Tc2]  "B12_r_B12Tc2"
  Bc2_r_Bc2B12/1 -> [rBc2B12]  "Bc2_r_Bc2B12"
  [rTc2P22] -> Bus Creator/1  "Tc2_r_Tc2P22"
  [rBc2B12] -> Bus Creator/6  "Bc2_r_Bc2B12"
  [rB12Tc2] -> Bus Creator/5  "B12_r_B12Tc2"
  [rBc2B32] -> Bus Creator/4  "Bc2_r_Bc2B32"
  [rB32B42] -> Bus Creator/3  "B32_r_B32B42"
  [rB42Tc2] -> Bus Creator/2  "B42_r_B42Tc2"
  Bus Creator/1 -> [PosVecsS2R]  "PosVecs_S2R"
  [PosVecsS2R] -> PosVecs_S2/1

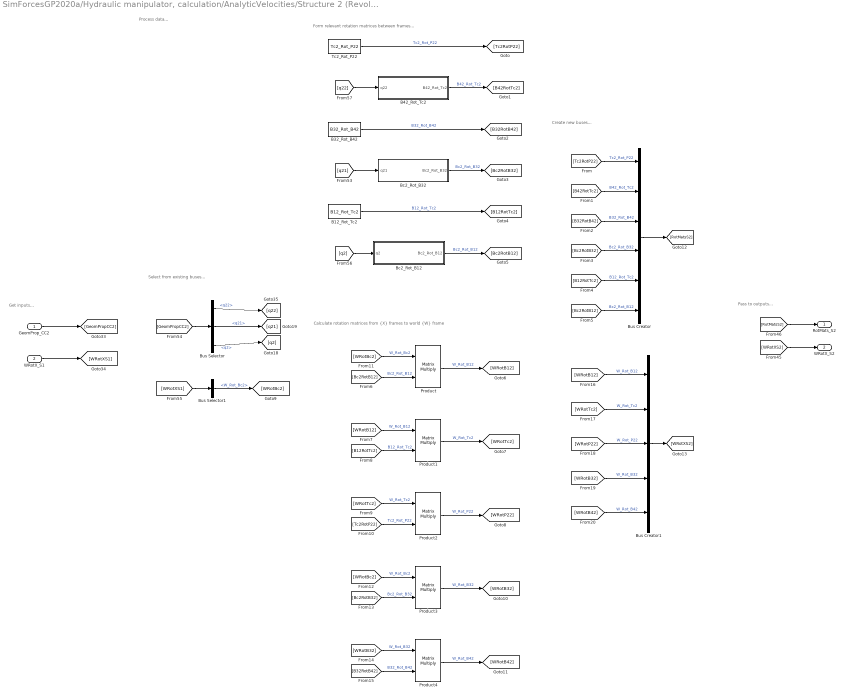
== system SimForcesGP2020a/Hydraulic manipulator, calculation/AnalyticVelocities/Structure 2 (Revolute segment)/RotMatsS2R ==
  note: Pass to outputs...
  note: Get inputs...
  note: Process data...
  note: Form relevant rotation matrices between frames...
  note: Create new buses...
  note: Select from existing buses...
  note: Calculate rotation matrices from {X} frames to world {W} frame
  GeomProp_CC2 : Inport
  WRotX_S1 : Inport  Port=2
  B12_Rot_Tc2 : Constant  Value=B12_Rot_Tc2
  B32_Rot_B42 : Constant  Value=B32_Rot_B42
  B42_Rot_Tc2 : MATLAB Function  TreatAsAtomicUnit=on
  Bc2_Rot_B12 : MATLAB Function  TreatAsAtomicUnit=on
  Bc2_Rot_B32 : MATLAB Function  TreatAsAtomicUnit=on
  Bus Creator : BusCreator  Inputs=Tc2_Rot_P22,B42_Rot_Tc2,B32_Rot_B42,Bc2_Rot_B32,B12_Rot_Tc2,Bc2_Rot_B12
  Bus Creator1 : BusCreator  Inputs=W_Rot_B12,W_Rot_Tc2,W_Rot_P22,W_Rot_B32,W_Rot_B42
  Bus Selector : BusSelector  OutputSignals=q22,q21,q2
  Bus Selector1 : BusSelector  OutputSignals=W_Rot_Bc2
  Product{,1..4} (5 alike) : Product  Multiplication=Matrix(*)
  Tc2_Rot_P22 : Constant  Value=Tc2_Rot_P22
  RotMats_S2 : Outport
  WRotX_S2 : Outport  Port=2
  wires:
  Bus Creator/1 -> [RotMatsS2]
  Tc2_Rot_P22/1 -> [Tc2RotP22]  "Tc2_Rot_P22"
  Bc2_Rot_B12/1(Bc2_Rot_B12) -> [Bc2RotB12]  "Bc2_Rot_B12"
  B12_Rot_Tc2/1 -> [B12RotTc2]  "B12_Rot_Tc2"
  Bc2_Rot_B32/1(Bc2_Rot_B32) -> [Bc2RotB32]  "Bc2_Rot_B32"
  B32_Rot_B42/1 -> [B32RotB42]  "B32_Rot_B42"
  B42_Rot_Tc2/1(B42_Rot_Tc2) -> [B42RotTc2]  "B42_Rot_Tc2"
  [Tc2RotP22] -> Bus Creator/1  "Tc2_Rot_P22"
  [B42RotTc2] -> Bus Creator/2  "B42_Rot_Tc2"
  [B32RotB42] -> Bus Creator/3  "B32_Rot_B42"
  [Bc2RotB32] -> Bus Creator/4  "Bc2_Rot_B32"
  [B12RotTc2] -> Bus Creator/5  "B12_Rot_Tc2"
  [Bc2RotB12] -> Bus Creator/6  "Bc2_Rot_B12"
  [Bc2RotB12] -> Product/2  "Bc2_Rot_B12"
  Product/1 -> [WRotB12]  "W_Rot_B12"
  [WRotB12] -> Product1/1  "W_Rot_B12"
  Product1/1 -> [WRotTc2]  "W_Rot_Tc2"
  [B12RotTc2] -> Product1/2  "B12_Rot_Tc2"
  [Tc2RotP22] -> Product2/2  "Tc2_Rot_P22"
  Product2/1 -> [WRotP22]  "W_Rot_P22"
  [WRotTc2] -> Product2/1  "W_Rot_Tc2"
  Bus Selector1/1 -> [WRotBc2]  "<W_Rot_Bc2>"
  [WRotBc2] -> Product/1  "W_Rot_Bc2"
  [WRotBc2] -> Product3/1  "W_Rot_Bc2"
  [Bc2RotB32] -> Product3/2  "Bc2_Rot_B32"
  Product3/1 -> [WRotB32]  "W_Rot_B32"
  Product4/1 -> [WRotB42]  "W_Rot_B42"
  [B32RotB42] -> Product4/2  "B32_Rot_B42"
  [WRotB32] -> Product4/1  "W_Rot_B32"
  [WRotB32] -> Bus Creator1/4  "W_Rot_B32"
  [WRotB42] -> Bus Creator1/5  "W_Rot_B42"
  [WRotP22] -> Bus Creator1/3  "W_Rot_P22"
  [WRotTc2] -> Bus Creator1/2  "W_Rot_Tc2"
  [WRotB12] -> Bus Creator1/1  "W_Rot_B12"
  Bus Creator1/1 -> [WRotXS2]
  [RotMatsS2] -> RotMats_S2/1
  [WRotXS2] -> WRotX_S2/1
  GeomProp_CC2/1 -> [GeomPropCC2]
  WRotX_S1/1 -> [WRotXS1]
  [WRotXS1] -> Bus Selector1/1
  [GeomPropCC2] -> Bus Selector/1
  Bus Selector/3 -> [q2]  "<q2>"
  Bus Selector/1 -> [q22]  "<q22>"
  Bus Selector/2 -> [q21]  "<q21>"
  [q21] -> Bc2_Rot_B32/1(q21)
  [q2] -> Bc2_Rot_B12/1(q2)
  [q22] -> B42_Rot_Tc2/1(q22)

== system SimForcesGP2020a/Hydraulic manipulator, calculation/AnalyticVelocities/Structure 2 (Revolute segment)/UMatS2R ==
  note: Pass to outputs...
  note: Process data...
  note: Create new buses...
  note: Get inputs...
  note: Select from existing buses...
  PosVecs_S2 : Inport
  RotMats_S2 : Inport  Port=2
  B12_U_Tc2 : MATLAB Function  TreatAsAtomicUnit=on
  B32_U_B42 : MATLAB Function  TreatAsAtomicUnit=on
  B42_U_Tc2 : MATLAB Function  TreatAsAtomicUnit=on
  Bc2_U_B12 : MATLAB Function  TreatAsAtomicUnit=on
  Bc2_U_B32 : MATLAB Function  TreatAsAtomicUnit=on
  Bus Creator : BusCreator  Inputs=Tc2_U_P22,B42_U_Tc2,B32_U_B42,Bc2_U_B32,B12_U_Tc2,Bc2_U_B12
  Bus Selector : BusSelector  OutputSignals=Tc2_r_Tc2P22,B42_r_B42Tc2,B32_r_B32B42,Bc2_r_Bc2B32,B12_r_B12Tc2,Bc2_r_Bc2B12
  Bus Selector1 : BusSelector  OutputSignals=Tc2_Rot_P22,B42_Rot_Tc2,B32_Rot_B42,Bc2_Rot_B32,B12_Rot_Tc2,Bc2_Rot_B12
  Tc2_U_P22 : MATLAB Function  TreatAsAtomicUnit=on
  UMatS2 : Outport
  wires:
  [B42RotTc2] -> B42_U_Tc2/2(B42_Rot_Tc2)
  [B32RotB42] -> B32_U_B42/2(B32_Rot_B42)
  [Bc2RotB32] -> Bc2_U_B32/2(Bc2_Rot_B32)
  [B12RotTc2] -> B12_U_Tc2/2(B12_Rot_Tc2)
  [Bc2RotB12] -> Bc2_U_B12/2(Bc2_Rot_B12)
  Bus Selector1/6 -> [Bc2RotB12]  "<Bc2_Rot_B12>"
  Bus Selector1/5 -> [B12RotTc2]  "<B12_Rot_Tc2>"
  Bus Selector1/4 -> [Bc2RotB32]  "<Bc2_Rot_B32>"
  Bus Selector1/3 -> [B32RotB42]  "<B32_Rot_B42>"
  Bus Selector1/2 -> [B42RotTc2]  "<B42_Rot_Tc2>"
  [rB32B42] -> B32_U_B42/1(B32_r_B32B42)
  [rBc2B32] -> Bc2_U_B32/1(Bc2_r_Bc2B32)
  [rB12Tc2] -> B12_U_Tc2/1(B12_r_B12Tc2)
  [rBc2B12] -> Bc2_U_B12/1(Bc2_r_Bc2B12)
  Bus Selector/6 -> [rBc2B12]  "<Bc2_r_Bc2B12>"
  Bus Selector/4 -> [rBc2B32]  "<Bc2_r_Bc2B32>"
  Bus Selector/5 -> [rB12Tc2]  "<B12_r_B12Tc2>"
  Bus Selector/3 -> [rB32B42]  "<B32_r_B32B42>"
  [rB42Tc2] -> B42_U_Tc2/1(B42_r_B42Tc2)
  Bus Selector/2 -> [rB42Tc2]  "<B42_r_B42Tc2>"
  Bus Selector/1 -> [rTc2P22]  "<Tc2_r_Tc2P22>"
  Bus Selector1/1 -> [Tc2RotP22]  "<Tc2_Rot_P22>"
  [rTc2P22] -> Tc2_U_P22/1(Tc2_r_Tc2P22)
  [Tc2RotP22] -> Tc2_U_P22/2(Tc2_Rot_P22)
  PosVecs_S2/1 -> [PosVecsS2]
  RotMats_S2/1 -> [RotMatsS2]
  [PosVecsS2] -> Bus Selector/1  "PosVecsS2"
  [RotMatsS2] -> Bus Selector1/1  "RotMatsS2"
  Tc2_U_P22/1(Tc2_U_P22) -> [Tc2UP22]  "Tc2_U_P22"
  [Tc2UP22] -> Bus Creator/1  "Tc2_U_P22"
  B12_U_Tc2/1(B12_U_Tc2) -> [B12UTc2]  "B12_U_Tc2"
  Bc2_U_B32/1(Bc2_U_B32) -> [Bc2UB32]  "Bc2_U_B32"
  B32_U_B42/1(B32_U_B42) -> [B32UB42]  "B32_U_B42"
  B42_U_Tc2/1(B42_U_Tc2) -> [B42UTc2]  "B42_U_Tc2"
  Bc2_U_B12/1(Bc2_U_B12) -> [Bc2UB12]  "Bc2_U_B12"
  [B42UTc2] -> Bus Creator/2  "B42_U_Tc2"
  [B32UB42] -> Bus Creator/3  "B32_U_B42"
  [Bc2UB32] -> Bus Creator/4  "Bc2_U_B32"
  [B12UTc2] -> Bus Creator/5  "B12_U_Tc2"
  [Bc2UB12] -> Bus Creator/6  "Bc2_U_B12"
  Bus Creator/1 -> [UMatS2]  "UMats_S2"
  [UMatS2] -> UMatS2/1  "UMats_S2"

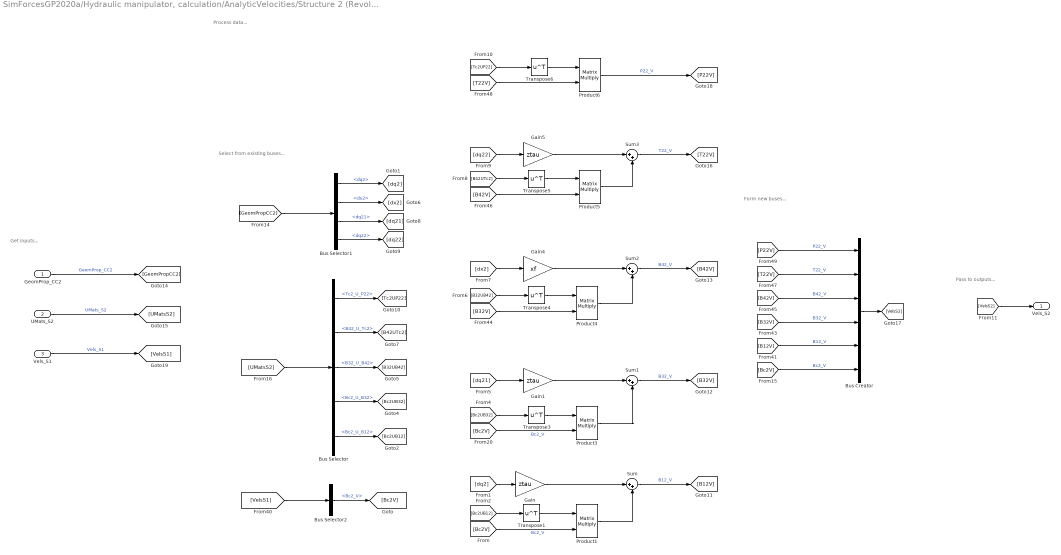
== system SimForcesGP2020a/Hydraulic manipulator, calculation/AnalyticVelocities/Structure 2 (Revolute segment)/VelsS2R ==
  note: Pass to outputs...
  note: Process data...
  note: Form new buses...
  note: Select from existing buses...
  note: Get inputs...
  GeomProp_CC2 : Inport
  UMats_S2 : Inport  Port=2
  Vels_S1 : Inport  Port=3
  Bus Creator : BusCreator  Inputs=P22_V,T22_V,B42_V,B32_V,B12_V,Bc2_V
  Bus Selector : BusSelector  OutputSignals=Tc2_U_P22,B42_U_Tc2,B32_U_B42,Bc2_U_B32,Bc2_U_B12
  Bus Selector1 : BusSelector  OutputSignals=dq2,dx2,dq21,dq22
  Bus Selector2 : BusSelector  OutputSignals=Bc2_V
  Gain : Gain  Gain=ztau
  Gain1 : Gain  Gain=ztau
  Gain4 : Gain  Gain=xf
  Gain5 : Gain  Gain=ztau
  Product{1,3..6} (5 alike) : Product  Multiplication=Matrix(*)
  Sum{,1..3} (4 alike) : Sum  Inputs=|++
  Transpose{1,3..6} (5 alike) : Math  Operator=transpose  SaturateOnIntegerOverflow=on
  Vels_S2 : Outport
  wires:
  [dq22] -> Gain5/1
  Bus Selector1/3 -> [dq21]  "<dq21>"
  Bus Selector1/4 -> [dq22]  "<dq22>"
  Transpose5/1 -> Product5/1
  [B42UTc2] -> Transpose5/1
  Bus Selector/2 -> [B42UTc2]  "<B42_U_Tc2>"
  [dx2] -> Gain4/1
  Bus Selector1/2 -> [dx2]  "<dx2>"
  Sum1/1 -> [B32V]  "B32_V"
  [B32UB42] -> Transpose4/1
  Transpose4/1 -> Product4/1
  Bus Selector/3 -> [B32UB42]  "<B32_U_B42>"
  [dq21] -> Gain1/1
  Product3/1 -> Sum1/2
  [Bc2UB32] -> Transpose3/1
  Transpose3/1 -> Product3/1
  Bus Selector/4 -> [Bc2UB32]  "<Bc2_U_B32>"
  [Bc2UB12] -> Transpose1/1
  Bus Selector/5 -> [Bc2UB12]  "<Bc2_U_B12>"
  [dq2] -> Gain/1
  Bus Selector1/1 -> [dq2]  "<dq2>"
  Transpose1/1 -> Product1/1
  Product5/1 -> Sum3/2
  Gain4/1 -> Sum2/1
  Product4/1 -> Sum2/2
  Gain/1 -> Sum/1
  Gain5/1 -> Sum3/1
  Gain1/1 -> Sum1/1
  Sum/1 -> [B12V]  "B12_V"
  Product1/1 -> Sum/2
  Bus Selector2/1 -> [Bc2V]  "<Bc2_V>"
  Bus Selector/1 -> [Tc2UP22]  "<Tc2_U_P22>"
  Transpose6/1 -> Product6/1
  [Tc2UP22] -> Transpose6/1
  GeomProp_CC2/1 -> [GeomPropCC2]  "GeomProp_CC2"
  UMats_S2/1 -> [UMatsS2]  "UMats_S2"
  Vels_S1/1 -> [VelsS1]  "Vels_S1"
  [VelsS1] -> Bus Selector2/1
  [UMatsS2] -> Bus Selector/1
  [GeomPropCC2] -> Bus Selector1/1
  [Bc2V] -> Bus Creator/6  "Bc2_V"
  [Bc2V] -> Product1/2  "Bc2_V"
  [Bc2V] -> Product3/2  "Bc2_V"
  [B12V] -> Bus Creator/5  "B12_V"
  [B32V] -> Bus Creator/4  "B32_V"
  [B32V] -> Product4/2
  Sum2/1 -> [B42V]  "B42_V"
  [B42V] -> Product5/2
  [B42V] -> Bus Creator/3  "B42_V"
  Sum3/1 -> [T22V]  "T22_V"
  [T22V] -> Bus Creator/2  "T22_V"
  [T22V] -> Product6/2
  [P22V] -> Bus Creator/1  "P22_V"
  Bus Creator/1 -> [VelsS2]
  [VelsS2] -> Vels_S2/1
  Product6/1 -> [P22V]  "P22_V"

== system SimForcesGP2020a/Hydraulic manipulator, calculation/AnalyticVelocities/Structure 1/GeomPropS1/LiftPistonStroke ==
  note: Pass to outputs...
  note: Process data...
  note: Derive piston stroke from q1-angle value...
  note: Get inputs...
  q1[rad] : Inport
  LiftPistonStroke : Fcn  Expr=sqrt(L1*L1+L11*L11+2*L1*L11*cos(u))-x10
  x1[m] : Outport
  wires:
  q1[rad]/1 -> [q1]
  [q1] -> LiftPistonStroke/1
  LiftPistonStroke/1 -> [x1]
  [x1] -> x1[m]/1

== system SimForcesGP2020a/Hydraulic manipulator, calculation/AnalyticVelocities/Structure 1/GeomPropS1/Subsystem ==
  note: Pass to output...
  note: Process data...
  note: Get inputs...
  dq1 : Inport
  x1 : Inport  Port=2
  q1 : Inport  Port=3
  LiftPistonVelocity : MATLAB Function  TreatAsAtomicUnit=on
  dx1 : Outport
  wires:
  dq1/1 -> [dq1]
  [dq1] -> LiftPistonVelocity/1(dq1)
  x1/1 -> [x1]
  [x1] -> LiftPistonVelocity/2(x1)
  q1/1 -> [q1]
  [q1] -> LiftPistonVelocity/3(q1)
  LiftPistonVelocity/1(dx1) -> [dx1]  "dx1"
  [dx1] -> dx1/1

== system SimForcesGP2020a/Hydraulic manipulator, calculation/AnalyticVelocities/Structure 1/GeomPropS1/Subsystem1 ==
  note: Pass to outputs...
  note: Process data...
  note: Get inputs...
  x1 : Inport
  q11 : Inport  Port=2
  dx1 : Inport  Port=3
  q11AngularVelocity : MATLAB Function  TreatAsAtomicUnit=on
  dq11 : Outport
  wires:
  x1/1 -> [x1]
  q11/1 -> [q11]
  dx1/1 -> [dx1]
  [x1] -> q11AngularVelocity/1(x1)  "x1"
  [q11] -> q11AngularVelocity/2(q11)  "q11"
  [dx1] -> q11AngularVelocity/3(dx1)  "dx1"
  q11AngularVelocity/1(dq11) -> [dq11]  "dq11"
  [dq11] -> dq11/1

== system SimForcesGP2020a/Hydraulic manipulator, calculation/AnalyticVelocities/Structure 1/GeomPropS1/Subsystem2 ==
  note: Process data...
  note: Pass to outputs...
  note: Get inputs...
  x1 : Inport
  q12 : Inport  Port=2
  dx1 : Inport  Port=3
  q12AngularVelocity : MATLAB Function  TreatAsAtomicUnit=on
  dq12 : Outport
  wires:
  dx1/1 -> [dx1]
  q12/1 -> [q12]
  [dq12] -> dq12/1
  q12AngularVelocity/1(dq12) -> [dq12]  "dq12"
  x1/1 -> [x1]
  [q12] -> q12AngularVelocity/2(q12)  "q12"
  [x1] -> q12AngularVelocity/1(x1)  "x1"
  [dx1] -> q12AngularVelocity/3(dx1)  "dx1"

== system SimForcesGP2020a/Hydraulic manipulator, calculation/AnalyticVelocities/Structure 1/GeomPropS1/q11-angle ==
  note: Pass to outputs...
  note: Process data...
  note: Get inputs...
  x1 : Inport
  Fcn : Fcn  Expr=-acos((L11*L11-(u+x10)*(u+x10)-L1*L1)/(-2*(u+x10)*L1))
  q11 : Outport
  wires:
  x1/1 -> [x1]
  [x1] -> Fcn/1
  Fcn/1 -> [q11]
  [q11] -> q11/1

== system SimForcesGP2020a/Hydraulic manipulator, calculation/AnalyticVelocities/Structure 1/GeomPropS1/q12-angle ==
  note: Pass to outputs...
  note: Process data...
  note: Get inputs...
  x1 : Inport
  Fcn : Fcn  Expr=-acos((L1*L1-(u+x10)*(u+x10)-L11*L11)/(-2*(u+x10)*L11))
  q12 : Outport
  wires:
  x1/1 -> [x1]
  [x1] -> Fcn/1
  Fcn/1 -> [q12]
  [q12] -> q12/1

== system SimForcesGP2020a/Hydraulic manipulator, calculation/AnalyticVelocities/Structure 1/GeomPropS1/q1Derivative ==
  note: Pass to outputs...
  note: Process data...
  note: Get inputs...
  q1 : Inport
  Derivative4 : Derivative
  dq1 : Outport
  wires:
  q1/1 -> [q1]  "q1"
  [q1] -> Derivative4/1  "q1"
  [dq1] -> dq1/1
  Derivative4/1 -> [dq1]  "dq1"

== system SimForcesGP2020a/Hydraulic manipulator, calculation/AnalyticVelocities/Structure 2 (Revolute segment)/GeomPropS2R/Subsystem4 ==
  note: Pass to outputs...
  note: Process data...
  note: Get inputs...
  x2 : Inport
  q21 : Inport  Port=2
  dx2 : Inport  Port=3
  q21AngularVelocity : MATLAB Function  TreatAsAtomicUnit=on
  dq21 : Outport
  wires:
  x2/1 -> [x2]  "x2"
  q21/1 -> [q21]  "q21"
  dx2/1 -> [dx2]  "dx2"
  [x2] -> q21AngularVelocity/1(x2)  "x2"
  q21AngularVelocity/1(dq21) -> [dq21]  "dq21"
  [dq21] -> dq21/1  "dq21"
  [dx2] -> q21AngularVelocity/2(dx2)  "dx2"
  [q21] -> q21AngularVelocity/3(q21)  "q21"

== system SimForcesGP2020a/Hydraulic manipulator, calculation/AnalyticVelocities/Structure 2 (Revolute segment)/GeomPropS2R/Subsystem5 ==
  note: Process data...
  note: Pass to outputs...
  note: Get inputs...
  x2 : Inport
  q22 : Inport  Port=2
  dx2 : Inport  Port=3
  q22AngularVelocity : MATLAB Function  TreatAsAtomicUnit=on
  dq22 : Outport
  wires:
  dx2/1 -> [dx2]  "dx2"
  q22/1 -> [q22]  "q22"
  [dq22] -> dq22/1  "dq22"
  q22AngularVelocity/1(dq22) -> [dq22]  "dq22"
  x2/1 -> [x2]  "x2"
  [x2] -> q22AngularVelocity/1(x2)  "x2"
  [dx2] -> q22AngularVelocity/2(dx2)  "dx2"
  [q22] -> q22AngularVelocity/3(q22)  "q22"

== system SimForcesGP2020a/Hydraulic manipulator, calculation/AnalyticVelocities/Structure 2 (Revolute segment)/GeomPropS2R/TiltPistonStroke ==
  note: Process data...
  note: Derive the tilt piston stroke from q2-angle value...
  note: Get inputs...
  note: Pass to outputs...
  q2[rad] : Inport
  TiltPistonStroke : Fcn  Expr=sqrt(L2*L2+L12*L12+2*L2*L12*cos(u))-x20
  x2[m] : Outport
  wires:
  [q2] -> TiltPistonStroke/1
  TiltPistonStroke/1 -> [x2]
  [x2] -> x2[m]/1
  q2[rad]/1 -> [q2]
